simulink library "visionmorphops"  (R2024b)
settings: Solver=ode45  StartTime=0.0  StopTime=10.0  RelTol=1e-3
undefined symbols (not defined in the file or in its folder): nhdims, nhood, strel
libraries: $bdroot x2
settings Model: Creator=The MathWorks, Inc.  LastModifiedBy=The MathWorks, Inc.
settings SolverCC: AlgebraicLoopSolver=TrustRegion
settings DataIOCC: LimitDataPoints=on  SaveFormat=Array  SignalLoggingSaveFormat=ModelDataLogs  ReturnWorkspaceOutputs=off
settings OptimizationCC: BlockReduction=off  BooleanDataType=off  LifeSpan=inf
settings DebuggingCC: SaveWithParameterizedLinksMsg=none  UnderspecifiedInitializationDetection=Classic  MergeDetectMultiDrivingBlocksExec=none  SignalResolutionControl=TryResolveAllWithWarning  UnconnectedInputMsg=warning  UnconnectedOutputMsg=warning  UnconnectedLineMsg=warning  SFUnexpectedBacktrackingDiag=warning  SFNoUnconditionalDefaultTransitionDiag=warning  SFExecutionAtInitializationDiag=none  ArithmeticOperatorsInVariantConditions=warning
settings HardwareCC: ProdBitPerPointer=32  ProdBitPerSizeT=32  ProdBitPerPtrDiffT=32  ProdLargestAtomicFloat=None  ProdIntDivRoundTo=Undefined  ProdEndianess=Unspecified  ProdWordSize=32  ProdHWDeviceType=32-bit Generic  TargetUnknown=on
settings ModelReferenceCC: EnableRefExpFcnMdlSchedulingChecks=on  PropagateSignalLabelsOutOfModel=off
settings SFSimCC: SimUseLocalCustomCode=off  SimGenImportedTypeDefs=on  CustomCodeUndefinedFunction=UseInterfaceOnly
settings RTWCC: RTWUseLocalCustomCode=off  GPUComputeCapability=3.5  DLArmComputeVersion=19.05
settings CodeAppCC: StateflowObjectComments=on
settings GRTTargetCC: TargetLangStandard=C89/C90 (ANSI)
settings ConfigComp: CovMetricSettings=dw  CovSaveCumulativeToWorkspaceVar=on  CovSaveSingleToWorkspaceVar=on  CovExternalEMLEnable=off

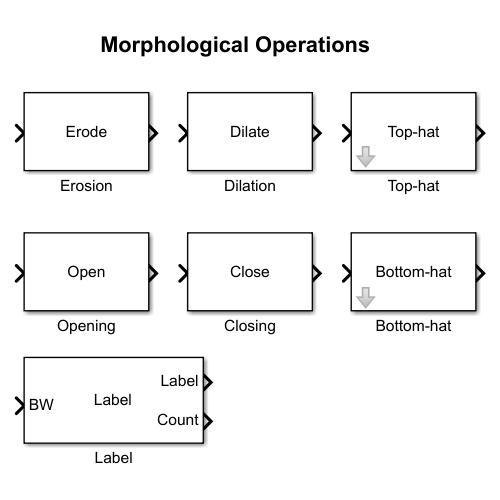
[thumbnail: Simulink's stored preview of the top-level diagram]
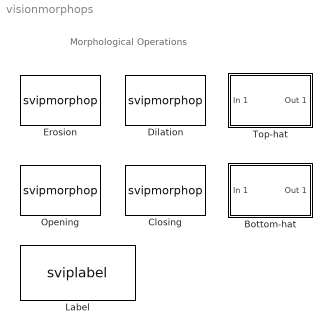
== system visionmorphops ==
  note: Morphological Operations
  Bottom-hat : Subsystem  mask(Bottom-hat){imgtype=Intensity, nhoodsrc=Specify via dialog, strel=strel('octagon',15)}
      mask prompts: imgtype "vision:masks:InputImageType"; nhoodsrc "vision:masks:NeighborhoodOrStructuringElementSrc"; strel "vision:masks:NeighborhoodOrStructuringElement"
      mask help: vision:masks:BottomHatDescription
      mask init:
      | nhoodsrc_str = get_param(gcbh,'nhoodsrc');
      | imgtype_str  = get_param(gcbh,'imgtype');
      | if strncmp(nhoodsrc_str,'Specify',5)
      | 	[si(1:2).port] = deal(1,1);
      | 	[si(1:2).txt] = deal('','');
      | else
      | 	[si(1:2).port] = deal(1,2);
      | 	if strncmp(imgtype_str,'Bina',4)
      | 		[si(1:2).txt] = deal('BW','Nhood');
      | 	else
      | 		[si(1:2).txt] = deal('I','Nhood');
      | 	end
      | end
      | 
      | vipblkhatfilter('init')
      mask Help: eval('visionblockhelp');
      mask TypeOptions imgtype: vision:masks:Intensity | vision:masks:Binary
      mask TypeOptions nhoodsrc: vision:masks:SpecifyViaDialog | vision:masks:InputPort
      mask Callback nhoodsrc: vipblkhatfilter
      mask Display:
      | disp('Bottom-hat')
      | port_label('input',si(1).port, si(1).txt);
      | port_label('input',si(2).port, si(2).txt);
  Closing : S-Function  FunctionName=svipmorphop  Parameters=3,nhoodsrc,nhood,nhdims  SFunctionDeploymentMode=off  EnableBusSupport=on  mask(Closing){nhoodsrc=Specify via dialog, strel=strel('line',5,45)}
      mask prompts: nhoodsrc "vision:masks:NeighborhoodOrStructuringElementSrc"; strel "vision:masks:NeighborhoodOrStructuringElement"
      mask help: vision:masks:ClosingDescription
      mask init:
      | nhoodsrc_str = get_param(gcbh,'nhoodsrc');
      | if strncmp(nhoodsrc_str,'Specify',5)
      | 	[si(1:2).port] = deal(1,1);
      | 	[si(1:2).txt] = deal('','');
      | else
      | 	[si(1:2).port] = deal(1,2);
      | 	[si(1:2).txt] = deal('I','Nhood');
      | end
      | [nhood nhdims] = vipblkmorphop(strel);
      mask Help: eval('visionblockhelp');
      mask TypeOptions nhoodsrc: vision:masks:SpecifyViaDialog | vision:masks:InputPort
      mask Callback nhoodsrc: vipblkmorphop
      mask Display:
      | disp('Close');
      | port_label('input',si(1).port, si(1).txt);
      | port_label('input',si(2).port, si(2).txt);
  Dilation : S-Function  FunctionName=svipmorphop  Parameters=1,nhoodsrc,nhood,nhdims  SFunctionDeploymentMode=off  EnableBusSupport=on  mask(Dilation){nhoodsrc=Specify via dialog, strel=[1 1; 1 1]}
      mask prompts: nhoodsrc "vision:masks:NeighborhoodOrStructuringElementSrc"; strel "vision:masks:NeighborhoodOrStructuringElement"
      mask help: vision:masks:DilationDescription
      mask init: same as visionmorphops/Closing
      mask Help: eval('visionblockhelp');
      mask TypeOptions nhoodsrc: vision:masks:SpecifyViaDialog | vision:masks:InputPort
      mask Callback nhoodsrc: vipblkmorphop
      mask Display:
      | disp('Dilate');
      | port_label('input',si(1).port, si(1).txt);
      | port_label('input',si(2).port, si(2).txt);
  Erosion : S-Function  FunctionName=svipmorphop  Parameters=0,nhoodsrc,nhood,nhdims  SFunctionDeploymentMode=off  EnableBusSupport=on  mask(Erosion){nhoodsrc=Specify via dialog, strel=strel('square',4)}
      mask prompts: nhoodsrc "vision:masks:NeighborhoodOrStructuringElementSrc"; strel "vision:masks:NeighborhoodOrStructuringElement"
      mask help: vision:masks:ErosionDescription
      mask init:
      | nhoodsrc_str = get_param(gcbh,'nhoodsrc');
      | if strncmp(nhoodsrc_str,'Specify',5)
      | 	[si(1:2).port] = deal(1,1);
      | 	[si(1:2).txt] = deal('','');
      | else
      | 	[si(1:2).port] = deal(1,2);
      | 	[si(1:2).txt] = deal('I','Nhood');
      | end
      | [nhood nhdims] = vipblkmorphop(strel);
      mask Help: eval('visionblockhelp');
      mask TypeOptions nhoodsrc: vision:masks:SpecifyViaDialog | vision:masks:InputPort
      mask Callback nhoodsrc: vipblkmorphop
      mask Display:
      | disp('Erode');
      | port_label('input',si(1).port, si(1).txt);
      | port_label('input',si(2).port, si(2).txt);
  Label : S-Function  FunctionName=sviplabel  Parameters=conn,output,outType,lastLabel  SFunctionDeploymentMode=off  EnableBusSupport=off  mask(Label){conn=8, output=Label matrix and number of labels, outType=Automatic, lastLabel=maximum value of the output data type}
      mask prompts: conn "vision:masks:Connectivity"; output "vision:masks:Output1"; outType "vision:masks:OutputDataType"; lastLabel "vision:masks:IfLabelExceedsDataTypeSize"
      mask help: vision:masks:LabelDescription
      mask init:
      | output_str = get_param(gcbh,'output');
      | if strncmp(output_str,'Label matrix and',16)
      |     [so(1:2).port] = deal(1,2);
      |     [so(1:2).txt] = deal('Label','Count');
      | elseif strcmp(output_str,'Label matrix')
      |     [so(1:2).port] = deal(1,1);
      |     [so(1:2).txt] = deal('Label','Label');
      | else
      |     [so(1:2).port] = deal(1,1);
      |     [so(1:2).txt] = deal('Count','Count');
      | end
      mask Help: eval('visionblockhelp');
      mask TypeOptions conn: 8 | 4
      mask TypeOptions output: vision:masks:LabelMatrixAndNumberOfLabels | vision:masks:LabelMatrix | vision:masks:NumberOfLabels
      mask TypeOptions outType: vision:masks:Automatic | uint32 | uint16 | uint8
      mask Callback outType: vipblklabel
      mask TypeOptions lastLabel: vision:masks:MaximumValueOfTheOutputDataType | vision:masks:Zero
      mask Display:
      | disp('Label');
      | port_label('input',1,'BW');
      | port_label('output',so(1).port,so(1).txt);
      | port_label('output',so(2).port,so(2).txt);
  Opening : S-Function  FunctionName=svipmorphop  Parameters=2,nhoodsrc,nhood,nhdims  SFunctionDeploymentMode=off  EnableBusSupport=on  mask(Opening){nhoodsrc=Specify via dialog, strel=strel('disk',5)}
      mask prompts: nhoodsrc "vision:masks:NeighborhoodOrStructuringElementSrc"; strel "vision:masks:NeighborhoodOrStructuringElement"
      mask help: vision:masks:OpeningDescription
      mask init: same as visionmorphops/Erosion
      mask Help: eval('visionblockhelp');
      mask TypeOptions nhoodsrc: vision:masks:SpecifyViaDialog | vision:masks:InputPort
      mask Callback nhoodsrc: vipblkmorphop
      mask Display:
      | disp('Open');
      | port_label('input',si(1).port, si(1).txt);
      | port_label('input',si(2).port, si(2).txt);
  Top-hat : Subsystem  mask(Top-hat){imgtype=Intensity, nhoodsrc=Specify via dialog, strel=strel('square',4);}
      mask prompts: imgtype "vision:masks:InputImageType"; nhoodsrc "vision:masks:NeighborhoodOrStructuringElementSrc"; strel "vision:masks:NeighborhoodOrStructuringElement"
      mask help: vision:masks:TopHatDescription
      mask init:
      | nhoodsrc_str = get_param(gcbh,'nhoodsrc');
      | imgtype_str = get_param(gcbh,'imgtype');
      | if strncmp(nhoodsrc_str,'Specify',5)
      | 	[si(1:2).port] = deal(1,1);
      | 	[si(1:2).txt] = deal('','');
      | else
      | 	[si(1:2).port] = deal(1,2);
      | 	if strncmp(imgtype_str,'Bina',4)
      | 		[si(1:2).txt] = deal('BW','Nhood');
      | 	else
      | 		[si(1:2).txt] = deal('I','Nhood');
      | 	end
      | end
      | 
      | vipblkhatfilter('init');
      mask Help: eval('visionblockhelp');
      mask TypeOptions imgtype: vision:masks:Intensity | vision:masks:Binary
      mask TypeOptions nhoodsrc: vision:masks:SpecifyViaDialog | vision:masks:InputPort
      mask Callback nhoodsrc: vipblkhatfilter
      mask Display:
      | disp('Top-hat')
      | port_label('input',si(1).port, si(1).txt);
      | port_label('input',si(2).port, si(2).txt);

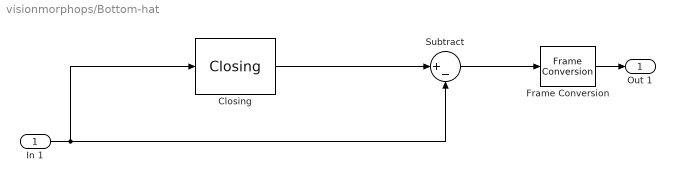
== system visionmorphops/Bottom-hat ==
  In 1 : Inport
  Closing : $bdroot/Closing  nhoodsrc=Specify via dialog  strel=strel
  Frame Conversion : FrameConversion  OutFrame=Sample-based
  Subtract : Sum  Inputs=|+-  InputSameDT=on  SaturateOnIntegerOverflow=on  OutDataTypeStr=Inherit: Same as first input
  Out 1 : Outport
  wires:
  In 1/1 -> Closing/1, Subtract/2
  Closing/1 -> Subtract/1
  Frame Conversion/1 -> Out 1/1
  Subtract/1 -> Frame Conversion/1

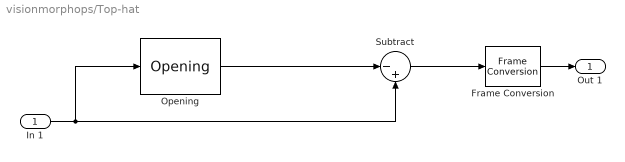
== system visionmorphops/Top-hat ==
  In 1 : Inport
  Frame Conversion : FrameConversion  OutFrame=Sample-based
  Opening : $bdroot/Opening  nhoodsrc=Specify via dialog  strel=strel
  Subtract : Sum  Inputs=|-+  InputSameDT=on  SaturateOnIntegerOverflow=on  OutDataTypeStr=Inherit: Same as first input
  Out 1 : Outport
  wires:
  In 1/1 -> Opening/1, Subtract/2
  Opening/1 -> Subtract/1
  Subtract/1 -> Frame Conversion/1
  Frame Conversion/1 -> Out 1/1
